simulink model "tanque2"  (R2022b)
settings: Solver=VariableStepAuto  StartTime=0.0  StopTime=300  RelTol=1e-3
model workspace (MAT data in the model file):
  Q1 = Simulink.Parameter
  Q1.Value = 34.77
  Q1.DataType = 'auto'
  Q1.Complexity = 'real'
  Q1.Dimensions = [1 1]
undefined symbols (not defined in the file or in its folder): a, b
settings Model: Creator=emmanuel  LastModifiedBy=emmanuel

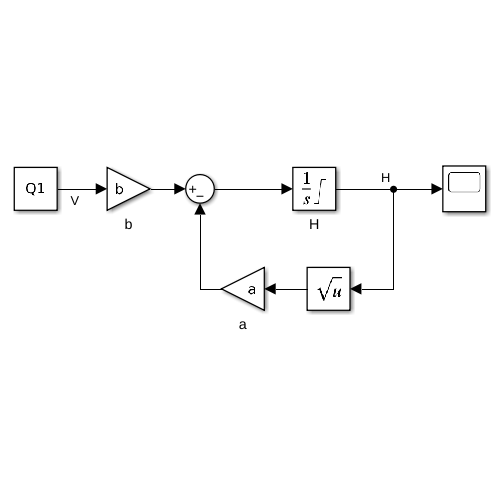
[thumbnail: Simulink's stored preview of the top-level diagram]
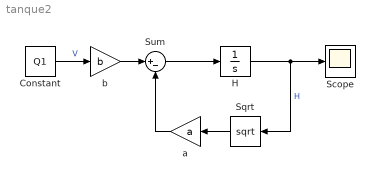
== system tanque2 ==
  Constant : Constant  Value=Q1
  H : Integrator  InitialCondition=0.5  LimitOutput=on  UpperSaturationLimit=3  LowerSaturationLimit=0
  Scope : Scope
  Sqrt : Sqrt
  Sum : Sum  Inputs=|+-  SaturateOnIntegerOverflow=on
  a : Gain  Gain=a  SaturateOnIntegerOverflow=on  OutDataTypeStr=Inherit: Same as input  ParamDataTypeStr=Inherit: Same as input
  b : Gain  Gain=b  SaturateOnIntegerOverflow=on  OutDataTypeStr=Inherit: Same as input  ParamDataTypeStr=Inherit: Same as input
  wires:
  H/1 -> Scope/1, Sqrt/1  "H"
  Constant/1 -> b/1  "V"
  b/1 -> Sum/1
  a/1 -> Sum/2
  Sqrt/1 -> a/1
  Sum/1 -> H/1
